simulink model "BatterySwitchingControl"  (R2024b)
settings: Solver=VariableStepAuto  StartTime=0.0  StopTime=10.0  RelTol=1e-3
libraries: spsIdealSwitchLib x4
settings Model: Creator=Nadir  LastModifiedBy=Nadir

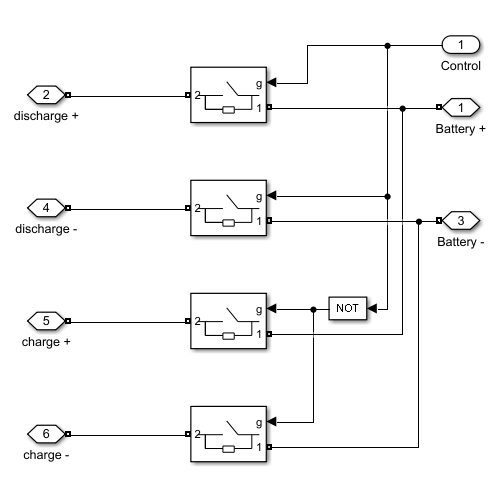
[thumbnail: Simulink's stored preview of the top-level diagram]
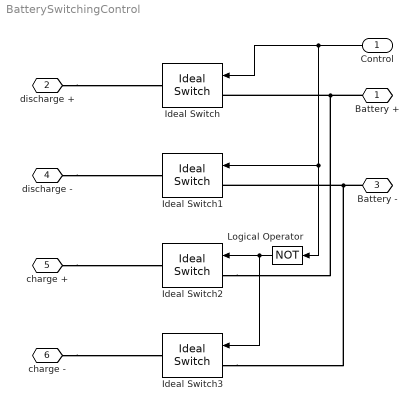
== system BatterySwitchingControl ==
  Control : Inport
  Ideal Switch{,1..3} (4 alike) : spsIdealSwitchLib/Ideal Switch  Ron=0.001  Lon=0  IC=0  Rs=1e5  Cs=inf  Measurements=off
  Logical Operator : Logic  Operator=NOT  AllPortsSameDT=off  OutDataTypeStr=boolean
  Battery + : PMIOPort  Side=Left
  discharge + : PMIOPort  Port=2  Side=Left
  Battery - : PMIOPort  Port=3  Side=Left
  discharge - : PMIOPort  Port=4  Side=Left
  charge + : PMIOPort  Port=5  Side=Left
  charge - : PMIOPort  Port=6  Side=Left
  wires:
  Control/1 -> Ideal Switch1/1, Logical Operator/1, Ideal Switch/1
  Logical Operator/1 -> Ideal Switch3/1, Ideal Switch2/1
  connections:
  discharge +/RConn1 -- Ideal Switch/RConn1
  discharge -/RConn1 -- Ideal Switch1/RConn1
  charge +/RConn1 -- Ideal Switch2/RConn1
  charge -/RConn1 -- Ideal Switch3/RConn1
  Battery +/RConn1 -- Ideal Switch2/LConn1 -- Ideal Switch/LConn1
  Battery -/RConn1 -- Ideal Switch3/LConn1 -- Ideal Switch1/LConn1
